simulink model "multi_fault_diagnostic_2600_12"  (R2020b)
settings: Solver=ode23tb  StartTime=0.0  StopTime=5433  MaxStep=0.1  RelTol=1e-3
undefined symbols (not defined in the file): Ion, Lithium
libraries: powerlib x30, electricdrivelib x12, simulink x2
settings Model: Creator=48572  LastModifiedBy=48572
settings DataIOCC: ReturnWorkspaceOutputs=off
settings DebuggingCC: ArithmeticOperatorsInVariantConditions=warning
settings SFSimCC: SimUseLocalCustomCode=off  CustomCodeUndefinedFunction=UseInterfaceOnly
settings RTWCC: RTWUseLocalCustomCode=off
settings CodeAppCC: StateflowObjectComments=on
settings SimscapeCC: SimscapeNormalizeSystem=off

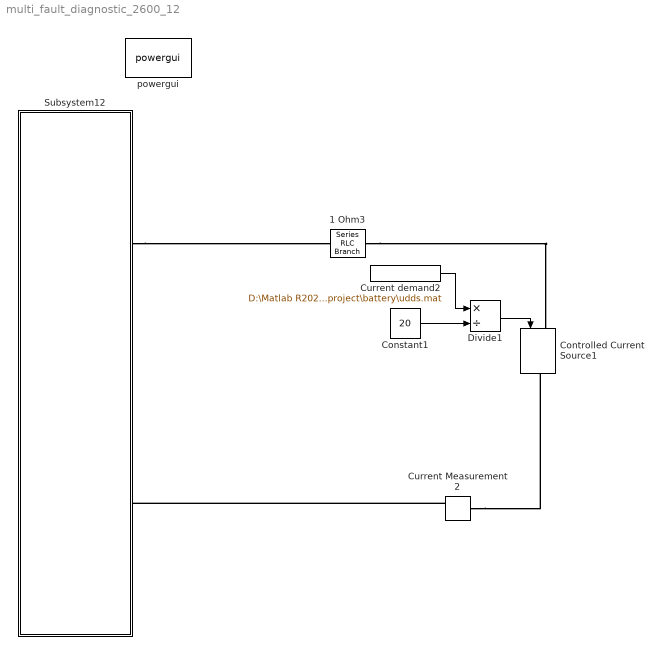
== system multi_fault_diagnostic_2600_12 ==
  1 Ohm3 : powerlib/Elements/Series RLC Branch  LConnTagsString=__new0  RConnTagsString=__new0  BranchType=R  Resistance=10000  Inductance=0.1  SetiL0=off  InitialCurrent=0  Capacitance=[]  Setx0=off  InitialVoltage=0  Measurements=None
  Constant1 : Constant  Value=20
  Controlled Current Source1 : powerlib/Electrical Sources/Controlled Current Source  Initialize=on  Source_Type=AC  Amplitude=0  Phase=0  Frequency=0  Measurements=None
  Current Measurement2 : powerlib/Measurements/Current Measurement  PhasorSimulation=off  OutputType=Complex  PSBequivalent=0
  Current demand2 : FromFile  FileName=D:\Matlab R2020b\project\battery\udds.mat  OutDataTypeStr=double  SampleTime=0
  Divide1 : Product  Inputs=*/
  Subsystem12 : Subsystem
  powergui : powerlib/powergui  Priority=1  SimulationMode=Continuous  SampleTime=50e-3  frequency=60  Iterations=50  frequencyindice=0  Pbase=100e6  ErrMax=1e-4  UnitsV=kV  UnitsW=MW  buscounter=0  FunctionMessages=off  echomessages=off  EnableUseOfTLC=off  CurrentSourceSwitches=off  DisableSnubberDevices=off  DisableRonSwitches=off  DisableVfSwitches=off  DisplayEquations=off  AutomaticDiscreteSolvers=off  SolverType=Tustin/Backward Euler (TBE)  Interpol=off  ExternalGateDelay=off  methode=off  Ts=10  x0status=blocks  SPID=off  SwTol=0  HookPort=off  NonlinearTolerance=1e-4  nMaxIteration=100  ContinueOnMaxIteration=off  RestoreLinks=warning  ResistiveCurrentMeasurement=off  Frange=[0:2:500]  Ylog=off  Xlog=on  ShowGrid=off  save=off  variable=ZData  structure=0  ZoomFFT=off  StartTime=0.0  cycles=1  DisplayStyle=1  fundamental=60  FreqAxis=off  MaxFrequency=1000  frequencyindicesteady=1  RmsSteady=1  display=off
  wires:
  Current demand2/1 -> Divide1/1
  Constant1/1 -> Divide1/2
  Divide1/1 -> Controlled Current Source1/1
  connections:
  Subsystem12/LConn1 -- 1 Ohm3/RConn1
  Current Measurement2/LConn1 -- Controlled Current Source1/RConn1
  1 Ohm3/LConn1 -- Controlled Current Source1/LConn1
  Current Measurement2/RConn1 -- Subsystem12/LConn2

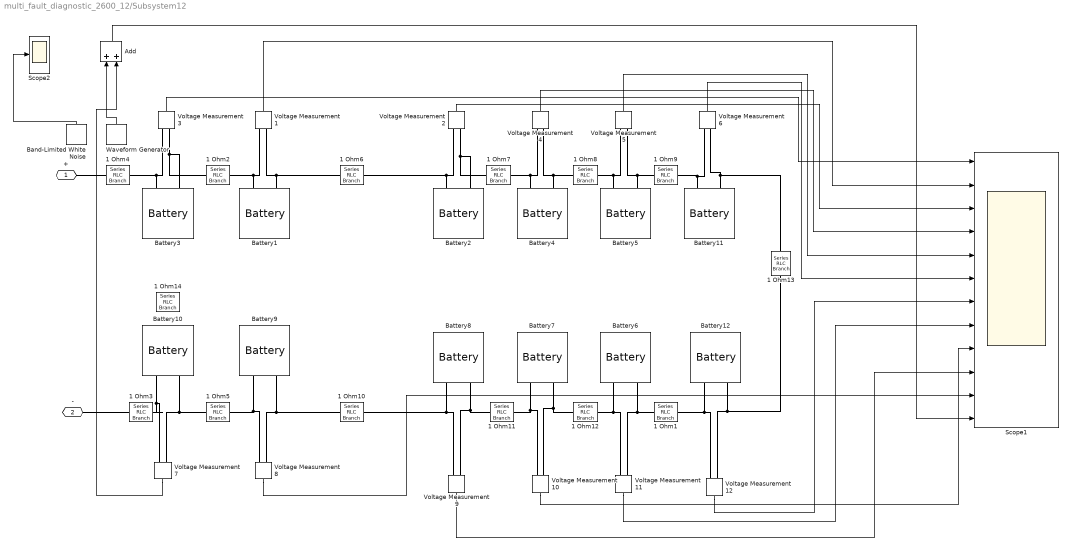
== system multi_fault_diagnostic_2600_12/Subsystem12 ==
  1 Ohm1 : powerlib/Elements/Series RLC Branch  LConnTagsString=__new0  RConnTagsString=__new0  BranchType=R  Resistance=0.012  Inductance=0.1  SetiL0=off  InitialCurrent=0  Capacitance=[]  Setx0=off  InitialVoltage=0  Measurements=None
  1 Ohm10 : powerlib/Elements/Series RLC Branch  LConnTagsString=__new0  RConnTagsString=__new0  BranchType=R  Resistance=0.02  Inductance=0.1  SetiL0=off  InitialCurrent=0  Capacitance=[]  Setx0=off  InitialVoltage=0  Measurements=None
  1 Ohm11 : powerlib/Elements/Series RLC Branch  LConnTagsString=__new0  RConnTagsString=__new0  BranchType=R  Resistance=0.023  Inductance=0.1  SetiL0=off  InitialCurrent=0  Capacitance=[]  Setx0=off  InitialVoltage=0  Measurements=None
  1 Ohm12 : powerlib/Elements/Series RLC Branch  LConnTagsString=__new0  RConnTagsString=__new0  BranchType=R  Resistance=0.070  Inductance=0.1  SetiL0=off  InitialCurrent=0  Capacitance=[]  Setx0=off  InitialVoltage=0  Measurements=None
  1 Ohm{2..4,6..9,13} (8 alike) : powerlib/Elements/Series RLC Branch  LConnTagsString=__new0  RConnTagsString=__new0  BranchType=R  Resistance=0.017  Inductance=0.1  SetiL0=off  InitialCurrent=0  Capacitance=[]  Setx0=off  InitialVoltage=0  Measurements=None
  1 Ohm14 : powerlib/Elements/Series RLC Branch  LConnTagsString=__new0  RConnTagsString=__new0  BranchType=R  Resistance=10  Inductance=0.1  SetiL0=off  InitialCurrent=0  Capacitance=[]  Setx0=off  InitialVoltage=0  Measurements=None
  1 Ohm5 : powerlib/Elements/Series RLC Branch  LConnTagsString=__new0  RConnTagsString=__new0  BranchType=R  Resistance=0.018  Inductance=0.1  SetiL0=off  InitialCurrent=0  Capacitance=[]  Setx0=off  InitialVoltage=0  Measurements=None
  Add : Sum
  Band-Limited White Noise : simulink/Sources/Band-Limited White Noise  Cov=[0.00001]  Ts=0.1  seed=[23341]
  Battery1 : electricdrivelib/Extra Sources/Battery  BatType=Lithium-Ion  ShowTempParam=off  ThermalPreset=no  ShowAgeParam=off  NomV=3.7  NomQ=2.6  SOC=99  Batt_Tr=30  PresetModel=off  MaxQ=2.6  MinV=2.775  FullV=4.3068  Dis_rate=0.58696  R=0.026407  Normal_OP=1.2209  expZone="[3.9974    0.066326]"  current=[6.5 13 32.5]  Units=Time  Tci=20  NomT=25  T2=0  MaxQ2=2.208  FullV2=3.45  Normal_OP2=2.8  expZone2="[3.22        0.23]"  Rca=0.6  ti=1000  Dp=0  Neq0=0  Tsim=1e6  Ta1=25  Qeol=5.4*0.9  Reol=0.013333*1.2  Char_age=[2.3478, 3]  Dis_age=[2.3478, 10]  N1=1500  N2=10500  N3=1000  N4=1400  Ta2=45  N5=950
  Battery10 : electricdrivelib/Extra Sources/Battery  BatType=Lithium-Ion  ShowTempParam=off  ThermalPreset=no  ShowAgeParam=off  NomV=3.7  NomQ=2.6  SOC=98  Batt_Tr=30  PresetModel=off  MaxQ=2.6  MinV=2.775  FullV=4.3068  Dis_rate=0.58696  R=0.028407  Normal_OP=1.2209  expZone="[3.9974    0.066326]"  current=[6.5 13 32.5]  Units=Time  Tci=20  NomT=25  T2=0  MaxQ2=2.208  FullV2=3.45  Normal_OP2=2.8  expZone2="[3.22        0.23]"  Rca=0.6  ti=1000  Dp=0  Neq0=0  Tsim=1e6  Ta1=25  Qeol=5.4*0.9  Reol=0.013333*1.2  Char_age=[2.3478, 3]  Dis_age=[2.3478, 10]  N1=1500  N2=10500  N3=1000  N4=1400  Ta2=45  N5=950
  Battery11 : electricdrivelib/Extra Sources/Battery  BatType=Lithium-Ion  ShowTempParam=off  ThermalPreset=no  ShowAgeParam=off  NomV=3.7  NomQ=2.6  SOC=99  Batt_Tr=30  PresetModel=off  MaxQ=2.6  MinV=2.775  FullV=4.3068  Dis_rate=0.58696  R=0.028807  Normal_OP=1.2209  expZone="[3.9974    0.066326]"  current=[6.5 13 32.5]  Units=Time  Tci=20  NomT=25  T2=0  MaxQ2=2.208  FullV2=3.45  Normal_OP2=2.8  expZone2="[3.22        0.23]"  Rca=0.6  ti=1000  Dp=0  Neq0=0  Tsim=1e6  Ta1=25  Qeol=5.4*0.9  Reol=0.013333*1.2  Char_age=[2.3478, 3]  Dis_age=[2.3478, 10]  N1=1500  N2=10500  N3=1000  N4=1400  Ta2=45  N5=950
  Battery12 : electricdrivelib/Extra Sources/Battery  BatType=Lithium-Ion  ShowTempParam=off  ThermalPreset=no  ShowAgeParam=off  NomV=3.7  NomQ=2.6  SOC=99  Batt_Tr=30  PresetModel=off  MaxQ=2.6  MinV=2.775  FullV=4.3068  Dis_rate=0.58696  R=0.028407  Normal_OP=1.2209  expZone="[3.9974    0.066326]"  current=[6.5 13 32.5]  Units=Time  Tci=20  NomT=25  T2=0  MaxQ2=2.208  FullV2=3.45  Normal_OP2=2.8  expZone2="[3.22        0.23]"  Rca=0.6  ti=1000  Dp=0  Neq0=0  Tsim=1e6  Ta1=25  Qeol=5.4*0.9  Reol=0.013333*1.2  Char_age=[2.3478, 3]  Dis_age=[2.3478, 10]  N1=1500  N2=10500  N3=1000  N4=1400  Ta2=45  N5=950
  Battery2 : electricdrivelib/Extra Sources/Battery  BatType=Lithium-Ion  ShowTempParam=off  ThermalPreset=no  ShowAgeParam=off  NomV=3.7  NomQ=2.6  SOC=95  Batt_Tr=30  PresetModel=off  MaxQ=2.6  MinV=2.775  FullV=4.3068  Dis_rate=0.58696  R=0.026407  Normal_OP=1.2209  expZone="[3.9974    0.066326]"  current=[6.5 13 32.5]  Units=Time  Tci=20  NomT=25  T2=0  MaxQ2=2.208  FullV2=3.45  Normal_OP2=2.8  expZone2="[3.22        0.23]"  Rca=0.6  ti=1000  Dp=0  Neq0=0  Tsim=1e6  Ta1=25  Qeol=5.4*0.9  Reol=0.013333*1.2  Char_age=[2.3478, 3]  Dis_age=[2.3478, 10]  N1=1500  N2=10500  N3=1000  N4=1400  Ta2=45  N5=950
  Battery3 : electricdrivelib/Extra Sources/Battery  BatType=Lithium-Ion  ShowTempParam=off  ThermalPreset=no  ShowAgeParam=off  NomV=3.7  NomQ=2.6  SOC=97  Batt_Tr=30  PresetModel=off  MaxQ=2.6  MinV=2.775  FullV=4.3068  Dis_rate=0.58696  R=0.028407  Normal_OP=1.2209  expZone="[3.9974    0.066326]"  current=[6.5 13 32.5]  Units=Time  Tci=20  NomT=25  T2=0  MaxQ2=2.208  FullV2=3.45  Normal_OP2=2.8  expZone2="[3.22        0.23]"  Rca=0.6  ti=1000  Dp=0  Neq0=0  Tsim=1e6  Ta1=25  Qeol=5.4*0.9  Reol=0.013333*1.2  Char_age=[2.3478, 3]  Dis_age=[2.3478, 10]  N1=1500  N2=10500  N3=1000  N4=1400  Ta2=45  N5=950
  Battery4 : electricdrivelib/Extra Sources/Battery  BatType=Lithium-Ion  ShowTempParam=off  ThermalPreset=no  ShowAgeParam=off  NomV=3.7  NomQ=2.6  SOC=99  Batt_Tr=30  PresetModel=off  MaxQ=2.6  MinV=2.775  FullV=4.3068  Dis_rate=0.58696  R=0.0260507  Normal_OP=1.2209  expZone="[3.9974    0.066326]"  current=[6.5 13 32.5]  Units=Time  Tci=20  NomT=25  T2=0  MaxQ2=2.208  FullV2=3.45  Normal_OP2=2.8  expZone2="[3.22        0.23]"  Rca=0.6  ti=1000  Dp=0  Neq0=0  Tsim=1e6  Ta1=25  Qeol=5.4*0.9  Reol=0.013333*1.2  Char_age=[2.3478, 3]  Dis_age=[2.3478, 10]  N1=1500  N2=10500  N3=1000  N4=1400  Ta2=45  N5=950
  Battery5 : electricdrivelib/Extra Sources/Battery  BatType=Lithium-Ion  ShowTempParam=off  ThermalPreset=no  ShowAgeParam=off  NomV=3.7  NomQ=2.6  SOC=98  Batt_Tr=30  PresetModel=off  MaxQ=2.6  MinV=2.775  FullV=4.3068  Dis_rate=0.58696  R=0.028807  Normal_OP=1.2209  expZone="[3.9974    0.066326]"  current=[6.5 13 32.5]  Units=Time  Tci=20  NomT=25  T2=0  MaxQ2=2.208  FullV2=3.45  Normal_OP2=2.8  expZone2="[3.22        0.23]"  Rca=0.6  ti=1000  Dp=0  Neq0=0  Tsim=1e6  Ta1=25  Qeol=5.4*0.9  Reol=0.013333*1.2  Char_age=[2.3478, 3]  Dis_age=[2.3478, 10]  N1=1500  N2=10500  N3=1000  N4=1400  Ta2=45  N5=950
  Battery6 : electricdrivelib/Extra Sources/Battery  BatType=Lithium-Ion  ShowTempParam=off  ThermalPreset=no  ShowAgeParam=off  NomV=3.7  NomQ=2.6  SOC=99  Batt_Tr=30  PresetModel=off  MaxQ=2.6  MinV=2.775  FullV=4.3068  Dis_rate=0.58696  R=0.028407  Normal_OP=1.2209  expZone="[3.9974    0.066326]"  current=[6.5 13 32.5]  Units=Time  Tci=20  NomT=25  T2=0  MaxQ2=2.208  FullV2=3.45  Normal_OP2=2.8  expZone2="[3.22        0.23]"  Rca=0.6  ti=1000  Dp=0  Neq0=0  Tsim=1e6  Ta1=25  Qeol=5.4*0.9  Reol=0.013333*1.2  Char_age=[2.3478, 3]  Dis_age=[2.3478, 10]  N1=1500  N2=10500  N3=1000  N4=1400  Ta2=45  N5=950
  Battery7 : electricdrivelib/Extra Sources/Battery  BatType=Lithium-Ion  ShowTempParam=off  ThermalPreset=no  ShowAgeParam=off  NomV=3.7  NomQ=2.6  SOC=97  Batt_Tr=30  PresetModel=off  MaxQ=2.6  MinV=2.775  FullV=4.3068  Dis_rate=0.58696  R=0.028407  Normal_OP=1.2209  expZone="[3.9974    0.066326]"  current=[6.5 13 32.5]  Units=Time  Tci=20  NomT=25  T2=0  MaxQ2=2.208  FullV2=3.45  Normal_OP2=2.8  expZone2="[3.22        0.23]"  Rca=0.6  ti=1000  Dp=0  Neq0=0  Tsim=1e6  Ta1=25  Qeol=5.4*0.9  Reol=0.013333*1.2  Char_age=[2.3478, 3]  Dis_age=[2.3478, 10]  N1=1500  N2=10500  N3=1000  N4=1400  Ta2=45  N5=950
  Battery8 : electricdrivelib/Extra Sources/Battery  BatType=Lithium-Ion  ShowTempParam=off  ThermalPreset=no  ShowAgeParam=off  NomV=3.7  NomQ=2.6  SOC=98  Batt_Tr=30  PresetModel=off  MaxQ=2.6  MinV=2.775  FullV=4.3068  Dis_rate=0.58696  R=0.028407  Normal_OP=1.2209  expZone="[3.9974    0.066326]"  current=[6.5 13 32.5]  Units=Time  Tci=20  NomT=25  T2=0  MaxQ2=2.208  FullV2=3.45  Normal_OP2=2.8  expZone2="[3.22        0.23]"  Rca=0.6  ti=1000  Dp=0  Neq0=0  Tsim=1e6  Ta1=25  Qeol=5.4*0.9  Reol=0.013333*1.2  Char_age=[2.3478, 3]  Dis_age=[2.3478, 10]  N1=1500  N2=10500  N3=1000  N4=1400  Ta2=45  N5=950
  Battery9 : electricdrivelib/Extra Sources/Battery  BatType=Lithium-Ion  ShowTempParam=off  ThermalPreset=no  ShowAgeParam=off  NomV=3.7  NomQ=2.6  SOC=100  Batt_Tr=30  PresetModel=off  MaxQ=2.6  MinV=2.775  FullV=4.3068  Dis_rate=0.58696  R=0.028407  Normal_OP=1.2209  expZone="[3.9974    0.066326]"  current=[6.5 13 32.5]  Units=Time  Tci=20  NomT=25  T2=0  MaxQ2=2.208  FullV2=3.45  Normal_OP2=2.8  expZone2="[3.22        0.23]"  Rca=0.6  ti=1000  Dp=0  Neq0=0  Tsim=1e6  Ta1=25  Qeol=5.4*0.9  Reol=0.013333*1.2  Char_age=[2.3478, 3]  Dis_age=[2.3478, 10]  N1=1500  N2=10500  N3=1000  N4=1400  Ta2=45  N5=950
  Scope1 : Scope  NumInputPorts=12
  Scope2 : Scope
  Voltage Measurement{1..12} (12 alike) : powerlib/Measurements/Voltage Measurement  PhasorSimulation=off  OutputType=Complex  PSBequivalent=0
  Waveform Generator : simulink/Sources/Waveform Generator  OutMin=[]  OutMax=[]  OutDataTypeStr=double  SelectedSignal=1  Signals=sin('Amplitude', 0.1, 'Frequency', 0.01, 'Phase', 1)+sin('Amplitude', 0.1, 'Frequency', 0.02, 'Phase', 1)+sin('Amplitude', 0.1, 'Frequency', 0.05, 'Phase', 1)  BlockNames=MultiportSwitch_363e1a5791a74c1  SampleTime=0.1
  + : PMIOPort  Side=Left
  - : PMIOPort  Port=2  Side=Left
  wires:
  Voltage Measurement1/1 -> Scope1/2
  Voltage Measurement9/1 -> Scope1/10
  Voltage Measurement3/1 -> Scope1/1
  Waveform Generator/1 -> Add/1
  Voltage Measurement2/1 -> Scope1/3
  Voltage Measurement4/1 -> Scope1/4
  Voltage Measurement5/1 -> Scope1/5
  Voltage Measurement6/1 -> Scope1/6
  Voltage Measurement12/1 -> Scope1/7
  Voltage Measurement11/1 -> Scope1/8
  Voltage Measurement10/1 -> Scope1/9
  Voltage Measurement8/1 -> Scope1/11
  Add/1 -> Scope1/12
  Voltage Measurement7/1 -> Add/2
  Band-Limited White Noise/1 -> Scope2/1
  connections:
  Voltage Measurement2/LConn1 -- Battery2/LConn1 -- 1 Ohm6/LConn1
  Voltage Measurement3/LConn2 -- Battery3/LConn2 -- 1 Ohm2/RConn1
  Voltage Measurement4/LConn1 -- 1 Ohm7/LConn1 -- Battery4/LConn1
  Voltage Measurement5/LConn1 -- Battery5/LConn1 -- 1 Ohm8/LConn1
  Voltage Measurement2/LConn2 -- Battery2/LConn2 -- 1 Ohm7/RConn1
  Voltage Measurement4/LConn2 -- Battery4/LConn2 -- 1 Ohm8/RConn1
  Voltage Measurement1/LConn1 -- Battery1/LConn1 -- 1 Ohm2/LConn1
  Voltage Measurement1/LConn2 -- Battery1/LConn2 -- 1 Ohm6/RConn1
  1 Ohm4/RConn1 -- +/RConn1
  Voltage Measurement5/LConn2 -- Battery5/LConn2 -- 1 Ohm9/RConn1
  Voltage Measurement3/LConn1 -- Battery3/LConn1 -- 1 Ohm4/LConn1
  Voltage Measurement6/LConn1 -- 1 Ohm9/LConn1 -- Battery11/LConn1
  1 Ohm12/RConn1 -- Voltage Measurement10/LConn1 -- Battery7/LConn1
  1 Ohm12/LConn1 -- Voltage Measurement11/LConn2 -- Battery6/LConn2
  1 Ohm11/LConn1 -- Voltage Measurement10/LConn2 -- Battery7/LConn2
  1 Ohm1/RConn1 -- Voltage Measurement11/LConn1 -- Battery6/LConn1
  1 Ohm5/LConn1 -- Voltage Measurement8/LConn2 -- Battery9/LConn2
  -/RConn1 -- 1 Ohm3/RConn1
  1 Ohm11/RConn1 -- Voltage Measurement9/LConn1 -- Battery8/LConn1
  1 Ohm10/RConn1 -- Voltage Measurement8/LConn1 -- Battery9/LConn1
  1 Ohm10/LConn1 -- Voltage Measurement9/LConn2 -- Battery8/LConn2
  1 Ohm5/RConn1 -- Voltage Measurement7/LConn1 -- Battery10/LConn1
  1 Ohm3/LConn1 -- Voltage Measurement7/LConn2 -- Battery10/LConn2
  Voltage Measurement12/LConn1 -- 1 Ohm13/LConn1 -- Battery12/LConn1
  Battery12/LConn2 -- Voltage Measurement12/LConn2 -- 1 Ohm1/LConn1
  1 Ohm13/RConn1 -- Voltage Measurement6/LConn2 -- Battery11/LConn2
